simulink model "addition1"  (Simulink 5.0)
settings: Solver=ode45  StartTime=0.0  StopTime=10.0  RelTol=1e-3
libraries: fixpt_lib_4 x2
settings Model: Creator=svenhoffmann  LastModifiedBy=svenhoffmann  ExtModeAutoUpdateStatusClock=off

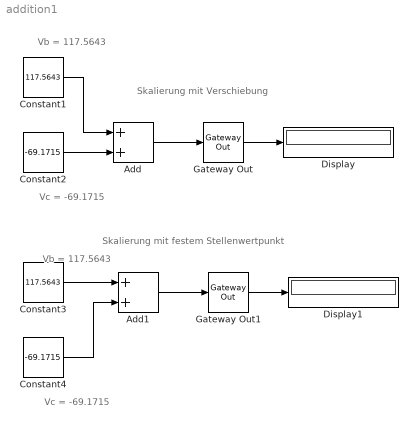
== system addition1 ==
  note: Skalierung mit Verschiebung
  note: Skalierung mit festem
      | Stellenwertpunkt
  note: Vb = 117.5643
  note: Vc = -69.1715
  note: Vc = -69.1715
  note: Vb = 117.5643
  Add : Sum  ShowAdditionalParam=on  OutDataTypeMode=Specify via dialog  OutScaling=[1.4742*2^-9, -24.2175]  RndMeth=Nearest
  Add1 : Sum  ShowAdditionalParam=on  OutDataTypeMode=Specify via dialog  OutScaling=2^-7  RndMeth=Ceiling
  Constant1 : Constant  Value=117.5643  ShowAdditionalParam=on  OutDataTypeMode=Specify via dialog  OutDataType=sfix(12)  OutScaling=[1.0513*2^-5, 59.6075]
  Constant2 : Constant  Value=-69.1715  ShowAdditionalParam=on  OutDataTypeMode=Specify via dialog  OutScaling=[1.474234375*2^-9, -83.8250]
  Constant3 : Constant  Value=117.5643  ShowAdditionalParam=on  OutDataTypeMode=Specify via dialog  OutDataType=sfix(12)  ConRadixGroup=Best Precision: Vector-wise  OutScaling=[1.0513*2^-5, 59.6075]
  Constant4 : Constant  Value=-69.1715  ShowAdditionalParam=on  OutDataTypeMode=Specify via dialog  ConRadixGroup=Best Precision: Vector-wise  OutScaling=[1.4742*2^-9, -83.8250]
  Display : Display
      settings: Format=short_e
  Display1 : Display
      settings: Format=short_e
  Gateway Out : fixpt_lib_4/Data Type/Gateway Out  OutRealWorld=Real World Value  OutBuiltInType=double  RndMeth=Nearest  DoSatur=off
  Gateway Out1 : fixpt_lib_4/Data Type/Gateway Out  OutRealWorld=Real World Value  OutBuiltInType=double  RndMeth=Nearest  DoSatur=on
  wires:
  Constant1/1 -> Add/1
  Constant2/1 -> Add/2
  Add/1 -> Gateway Out/1
  Gateway Out/1 -> Display/1
  Constant3/1 -> Add1/1
  Constant4/1 -> Add1/2
  Add1/1 -> Gateway Out1/1
  Gateway Out1/1 -> Display1/1
